simulink model "CrazyClover_Velocity_control"  (R2020b)
settings: Solver=VariableStepAuto  StartTime=0.0  StopTime=10.0  RelTol=1e-3
values from neighbouring files (symbols this model uses):
  controller_matrix = [mass/(4*gravity)*1000 mass/(4*gravity)*1000 mass/(4*gravity)*1000 mass/(4*gravity)*1000 ... (first row only)    [sim_param.m]
  kM1 = Armlength /sqrt(2)    [sim_param.m]
  kM2 = Armlength /sqrt(2)    [sim_param.m]
  kM3 = 1    [sim_param.m]
undefined symbols (not defined in the file or in its folder): Pitch, Pitchrate, Roll, Rollrate, Vel, Yaw, Yawrate
libraries: pid_lib x17
(part 2 of 2)

== system CrazyClover_Velocity_control/Controller/Subsystem3/Attitude PID/pitch PID ==
  u : Inport
  PID Controller1 : pid_lib/PID Controller  Controller=PID  Form=Parallel  TimeDomain=Continuous-time  UseExternalTs=off  SampleTime=-1  IntegratorMethod=Forward Euler  FilterMethod=Forward Euler  ControllerParametersSource=internal  P=0  I=Pitch.ki  D=0  UseFilter=on  N=100  TunerSelectOption=Transfer Function Based (PID Tuner App)  InitialConditionSource=internal  InitialConditionForIntegrator=0  InitialConditionForFilter=0  DifferentiatorICPrevScaledInput=0  ExternalReset=none  TrackingMode=off  Kt=1  LimitOutput=off  SatLimitsSource=internal  UpperSaturationLimit=inf  LowerSaturationLimit=-inf  LinearizeAsGain=on  AntiWindupMode=none  Kb=1  POutMin=[]  POutMax=[]  IOutMin=[]  IOutMax=[]  DOutMin=[]  DOutMax=[]  NOutMin=[]  NOutMax=[]  SumOutMin=[]  SumOutMax=[]  SaturationOutMin=[]  SaturationOutMax=[]  PParamMin=[]  PParamMax=[]  IParamMin=[]  IParamMax=[]  DParamMin=[]  DParamMax=[]  NParamMin=[]  NParamMax=[]  KbParamMin=[]  KbParamMax=[]  KtParamMin=[]  KtParamMax=[]  KbOutMin=[]  KbOutMax=[]  KtOutMin=[]  KtOutMax=[]  IntegratorOutMin=[]  IntegratorOutMax=[]  FilterOutMin=[]  FilterOutMax=[]  SumI1OutMin=[]  SumI1OutMax=[]  SumI2OutMin=[]  SumI2OutMax=[]  SumI3OutMin=[]  SumI3OutMax=[]  SumI4OutMin=[]  SumI4OutMax=[]  SumDOutMin=[]  SumDOutMax=[]  DifferentiatorOutMin=[]  DifferentiatorOutMax=[]  FilterDiffOutCoefMin=[]  FilterDiffOutCoefMax=[]  ReciprocalOutMin=[]  ReciprocalOutMax=[]  SumDenOutMin=[]  SumDenOutMax=[]  SumNumOutMin=[]  SumNumOutMax=[]  DivideOutMin=[]  DivideOutMax=[]  UdiffTsProdOutMin=[]  UdiffTsProdOutMax=[]  NTsProdOutMin=[]  NTsProdOutMax=[]  UintegralTsProdOutMin=[]  UintegralTsProdOutMax=[]  UngainTsProdOutMin=[]  UngainTsProdOutMax=[]  IntegratorContinuousStateAttributes=''  IntegratorStateMustResolveToSignalObject=off  IntegratorRTWStateStorageClass=Auto  FilterContinuousStateAttributes=''  FilterStateMustResolveToSignalObject=off  FilterRTWStateStorageClass=Auto  ParallelPVariant=InternalParameters  IdealPVariant=Disabled  IVariant=InternalParameters  DVariant=InternalParameters  IntegratorVariant=Continuous  SatVariant=Disabled  AWVariant=Passthrough  PCopyVariant=Disabled  TRVariant=Disabled  FdbkBlocksVariant=Forward  IdealPFdbkVariant=Disabled  SatFdbkVariant=Disabled  DerivativeFilterVariant=ContFilter  NVariant=InternalParameters  NCopyVariant=Disabled  FilterICVariant=InternalICsFilter  IntegratorICVariant=InternalICs  ExternalResetVariant=Disabled  TRSumVariant=Passthrough  SumFdbkVariant=Disabled  SumVariant=Sum_PID  TsampFilterVariant=InternalTs  TsampNgainVariant=Passthrough  TsampIntegralVariant=Passthrough  ExternalSaturationOutDataTypeStr=Inherit: Same as second input
  PID Controller2 : pid_lib/PID Controller  Controller=PID  Form=Parallel  TimeDomain=Continuous-time  UseExternalTs=off  SampleTime=-1  IntegratorMethod=Forward Euler  FilterMethod=Forward Euler  ControllerParametersSource=internal  P=Pitch.kp  I=0  D=0  UseFilter=on  N=100  TunerSelectOption=Transfer Function Based (PID Tuner App)  InitialConditionSource=internal  InitialConditionForIntegrator=0  InitialConditionForFilter=0  DifferentiatorICPrevScaledInput=0  ExternalReset=none  TrackingMode=off  Kt=1  LimitOutput=off  SatLimitsSource=internal  UpperSaturationLimit=inf  LowerSaturationLimit=-inf  LinearizeAsGain=on  AntiWindupMode=none  Kb=1  POutMin=[]  POutMax=[]  IOutMin=[]  IOutMax=[]  DOutMin=[]  DOutMax=[]  NOutMin=[]  NOutMax=[]  SumOutMin=[]  SumOutMax=[]  SaturationOutMin=[]  SaturationOutMax=[]  PParamMin=[]  PParamMax=[]  IParamMin=[]  IParamMax=[]  DParamMin=[]  DParamMax=[]  NParamMin=[]  NParamMax=[]  KbParamMin=[]  KbParamMax=[]  KtParamMin=[]  KtParamMax=[]  KbOutMin=[]  KbOutMax=[]  KtOutMin=[]  KtOutMax=[]  IntegratorOutMin=[]  IntegratorOutMax=[]  FilterOutMin=[]  FilterOutMax=[]  SumI1OutMin=[]  SumI1OutMax=[]  SumI2OutMin=[]  SumI2OutMax=[]  SumI3OutMin=[]  SumI3OutMax=[]  SumI4OutMin=[]  SumI4OutMax=[]  SumDOutMin=[]  SumDOutMax=[]  DifferentiatorOutMin=[]  DifferentiatorOutMax=[]  FilterDiffOutCoefMin=[]  FilterDiffOutCoefMax=[]  ReciprocalOutMin=[]  ReciprocalOutMax=[]  SumDenOutMin=[]  SumDenOutMax=[]  SumNumOutMin=[]  SumNumOutMax=[]  DivideOutMin=[]  DivideOutMax=[]  UdiffTsProdOutMin=[]  UdiffTsProdOutMax=[]  NTsProdOutMin=[]  NTsProdOutMax=[]  UintegralTsProdOutMin=[]  UintegralTsProdOutMax=[]  UngainTsProdOutMin=[]  UngainTsProdOutMax=[]  IntegratorContinuousStateAttributes=''  IntegratorStateMustResolveToSignalObject=off  IntegratorRTWStateStorageClass=Auto  FilterContinuousStateAttributes=''  FilterStateMustResolveToSignalObject=off  FilterRTWStateStorageClass=Auto  ParallelPVariant=InternalParameters  IdealPVariant=Disabled  IVariant=InternalParameters  DVariant=InternalParameters  IntegratorVariant=Continuous  SatVariant=Disabled  AWVariant=Passthrough  PCopyVariant=Disabled  TRVariant=Disabled  FdbkBlocksVariant=Forward  IdealPFdbkVariant=Disabled  SatFdbkVariant=Disabled  DerivativeFilterVariant=ContFilter  NVariant=InternalParameters  NCopyVariant=Disabled  FilterICVariant=InternalICsFilter  IntegratorICVariant=InternalICs  ExternalResetVariant=Disabled  TRSumVariant=Passthrough  SumFdbkVariant=Disabled  SumVariant=Sum_PID  TsampFilterVariant=InternalTs  TsampNgainVariant=Passthrough  TsampIntegralVariant=Passthrough  ExternalSaturationOutDataTypeStr=Inherit: Same as second input
  Saturation : Saturate  UpperLimit=Pitch.intupper  LowerLimit=Pitch.intlower
  Scope : Scope  NumInputPorts=2
  Sum : Sum  Inputs=|++
  y : Outport
  wires:
  Saturation/1 -> Scope/1, Sum/2
  PID Controller1/1 -> Saturation/1, Scope/2
  Sum/1 -> y/1
  u/1 -> PID Controller2/1, PID Controller1/1
  PID Controller2/1 -> Sum/1

== system CrazyClover_Velocity_control/Controller/Subsystem3/Attitude PID/roll PID ==
  u : Inport
  PID Controller1 : pid_lib/PID Controller  Controller=PID  Form=Parallel  TimeDomain=Continuous-time  UseExternalTs=off  SampleTime=-1  IntegratorMethod=Forward Euler  FilterMethod=Forward Euler  ControllerParametersSource=internal  P=0  I=Roll.ki  D=0  UseFilter=on  N=100  TunerSelectOption=Transfer Function Based (PID Tuner App)  InitialConditionSource=internal  InitialConditionForIntegrator=0  InitialConditionForFilter=0  DifferentiatorICPrevScaledInput=0  ExternalReset=none  TrackingMode=off  Kt=1  LimitOutput=off  SatLimitsSource=internal  UpperSaturationLimit=inf  LowerSaturationLimit=-inf  LinearizeAsGain=on  AntiWindupMode=none  Kb=1  POutMin=[]  POutMax=[]  IOutMin=[]  IOutMax=[]  DOutMin=[]  DOutMax=[]  NOutMin=[]  NOutMax=[]  SumOutMin=[]  SumOutMax=[]  SaturationOutMin=[]  SaturationOutMax=[]  PParamMin=[]  PParamMax=[]  IParamMin=[]  IParamMax=[]  DParamMin=[]  DParamMax=[]  NParamMin=[]  NParamMax=[]  KbParamMin=[]  KbParamMax=[]  KtParamMin=[]  KtParamMax=[]  KbOutMin=[]  KbOutMax=[]  KtOutMin=[]  KtOutMax=[]  IntegratorOutMin=[]  IntegratorOutMax=[]  FilterOutMin=[]  FilterOutMax=[]  SumI1OutMin=[]  SumI1OutMax=[]  SumI2OutMin=[]  SumI2OutMax=[]  SumI3OutMin=[]  SumI3OutMax=[]  SumI4OutMin=[]  SumI4OutMax=[]  SumDOutMin=[]  SumDOutMax=[]  DifferentiatorOutMin=[]  DifferentiatorOutMax=[]  FilterDiffOutCoefMin=[]  FilterDiffOutCoefMax=[]  ReciprocalOutMin=[]  ReciprocalOutMax=[]  SumDenOutMin=[]  SumDenOutMax=[]  SumNumOutMin=[]  SumNumOutMax=[]  DivideOutMin=[]  DivideOutMax=[]  UdiffTsProdOutMin=[]  UdiffTsProdOutMax=[]  NTsProdOutMin=[]  NTsProdOutMax=[]  UintegralTsProdOutMin=[]  UintegralTsProdOutMax=[]  UngainTsProdOutMin=[]  UngainTsProdOutMax=[]  IntegratorContinuousStateAttributes=''  IntegratorStateMustResolveToSignalObject=off  IntegratorRTWStateStorageClass=Auto  FilterContinuousStateAttributes=''  FilterStateMustResolveToSignalObject=off  FilterRTWStateStorageClass=Auto  ParallelPVariant=InternalParameters  IdealPVariant=Disabled  IVariant=InternalParameters  DVariant=InternalParameters  IntegratorVariant=Continuous  SatVariant=Disabled  AWVariant=Passthrough  PCopyVariant=Disabled  TRVariant=Disabled  FdbkBlocksVariant=Forward  IdealPFdbkVariant=Disabled  SatFdbkVariant=Disabled  DerivativeFilterVariant=ContFilter  NVariant=InternalParameters  NCopyVariant=Disabled  FilterICVariant=InternalICsFilter  IntegratorICVariant=InternalICs  ExternalResetVariant=Disabled  TRSumVariant=Passthrough  SumFdbkVariant=Disabled  SumVariant=Sum_PID  TsampFilterVariant=InternalTs  TsampNgainVariant=Passthrough  TsampIntegralVariant=Passthrough  ExternalSaturationOutDataTypeStr=Inherit: Same as second input
  PID Controller2 : pid_lib/PID Controller  Controller=PID  Form=Parallel  TimeDomain=Continuous-time  UseExternalTs=off  SampleTime=-1  IntegratorMethod=Forward Euler  FilterMethod=Forward Euler  ControllerParametersSource=internal  P=Roll.kp  I=0  D=0  UseFilter=on  N=100  TunerSelectOption=Transfer Function Based (PID Tuner App)  InitialConditionSource=internal  InitialConditionForIntegrator=0  InitialConditionForFilter=0  DifferentiatorICPrevScaledInput=0  ExternalReset=none  TrackingMode=off  Kt=1  LimitOutput=off  SatLimitsSource=internal  UpperSaturationLimit=inf  LowerSaturationLimit=-inf  LinearizeAsGain=on  AntiWindupMode=none  Kb=1  POutMin=[]  POutMax=[]  IOutMin=[]  IOutMax=[]  DOutMin=[]  DOutMax=[]  NOutMin=[]  NOutMax=[]  SumOutMin=[]  SumOutMax=[]  SaturationOutMin=[]  SaturationOutMax=[]  PParamMin=[]  PParamMax=[]  IParamMin=[]  IParamMax=[]  DParamMin=[]  DParamMax=[]  NParamMin=[]  NParamMax=[]  KbParamMin=[]  KbParamMax=[]  KtParamMin=[]  KtParamMax=[]  KbOutMin=[]  KbOutMax=[]  KtOutMin=[]  KtOutMax=[]  IntegratorOutMin=[]  IntegratorOutMax=[]  FilterOutMin=[]  FilterOutMax=[]  SumI1OutMin=[]  SumI1OutMax=[]  SumI2OutMin=[]  SumI2OutMax=[]  SumI3OutMin=[]  SumI3OutMax=[]  SumI4OutMin=[]  SumI4OutMax=[]  SumDOutMin=[]  SumDOutMax=[]  DifferentiatorOutMin=[]  DifferentiatorOutMax=[]  FilterDiffOutCoefMin=[]  FilterDiffOutCoefMax=[]  ReciprocalOutMin=[]  ReciprocalOutMax=[]  SumDenOutMin=[]  SumDenOutMax=[]  SumNumOutMin=[]  SumNumOutMax=[]  DivideOutMin=[]  DivideOutMax=[]  UdiffTsProdOutMin=[]  UdiffTsProdOutMax=[]  NTsProdOutMin=[]  NTsProdOutMax=[]  UintegralTsProdOutMin=[]  UintegralTsProdOutMax=[]  UngainTsProdOutMin=[]  UngainTsProdOutMax=[]  IntegratorContinuousStateAttributes=''  IntegratorStateMustResolveToSignalObject=off  IntegratorRTWStateStorageClass=Auto  FilterContinuousStateAttributes=''  FilterStateMustResolveToSignalObject=off  FilterRTWStateStorageClass=Auto  ParallelPVariant=InternalParameters  IdealPVariant=Disabled  IVariant=InternalParameters  DVariant=InternalParameters  IntegratorVariant=Continuous  SatVariant=Disabled  AWVariant=Passthrough  PCopyVariant=Disabled  TRVariant=Disabled  FdbkBlocksVariant=Forward  IdealPFdbkVariant=Disabled  SatFdbkVariant=Disabled  DerivativeFilterVariant=ContFilter  NVariant=InternalParameters  NCopyVariant=Disabled  FilterICVariant=InternalICsFilter  IntegratorICVariant=InternalICs  ExternalResetVariant=Disabled  TRSumVariant=Passthrough  SumFdbkVariant=Disabled  SumVariant=Sum_PID  TsampFilterVariant=InternalTs  TsampNgainVariant=Passthrough  TsampIntegralVariant=Passthrough  ExternalSaturationOutDataTypeStr=Inherit: Same as second input
  Saturation : Saturate  UpperLimit=Roll.intupper  LowerLimit=Roll.intlower
  Scope : Scope  NumInputPorts=2
  Sum : Sum  Inputs=|++
  y : Outport
  wires:
  PID Controller2/1 -> Sum/1
  u/1 -> PID Controller1/1, PID Controller2/1
  Sum/1 -> y/1
  PID Controller1/1 -> Scope/2, Saturation/1
  Saturation/1 -> Sum/2, Scope/1

== matlab function CrazyClover_Velocity_control/Controller/Subsystem3/velocity to attitude1 ==
  data: Vx input; Roll output; Pitch output; Vy input
function [Roll, Pitch]= fcn(Vx, Vy)

Roll = -Vy;
Pitch = +Vx;

== matlab function CrazyClover_Velocity_control/Plant/Subsystem/MATLAB Function ==
  data: R input; Rd output; Wb input
function Rd = fcn(R, Wb)
wx = Wb(1);
wy = Wb(2);
wz = Wb(3);
Wb = [ 0    -wz   wy;
       wz    0   -wx;
      -wy    wx   0];
Rd = R * Wb;

== matlab function CrazyClover_Velocity_control/Plant/actuator/pwm -> gram ==
  data: m1_pwm input; m1 output; m2_pwm input; m3_pwm input; m4_pwm input; m2 output; m3 output; m4 output
function [m1, m2,m3, m4]= func(m1_pwm, m2_pwm, m3_pwm, m4_pwm)

% F [16bit] Wddb [16bit]

% m1_pwm = moter_in(1);
% m2_pwm = moter_in(2);
% m3_pwm = moter_in(3);
% m4_pwm = moter_in(4);
m1_map = [2.1910e-07 0.0022 0];
m2_map = [2.1910e-07 0.0022 0];
m3_map = [2.1161e-07 0.0024 0];
m4_map = [2.0210e-07 0.0024 0];
% m_avs = (m1_pwm + m2_pwm + m3_pwm + m4_pwm)/4;
% m1_pwm = m_avs;
% m2_pwm = m_avs;
% m3_pwm = m_avs;
% m4_pwm = m_avs;
if m1_pwm > 0
    m1 = m1_map * [m1_pwm^2;m1_pwm;1];
else
    m1 = -m1_map * [m1_pwm^2;-m1_pwm;1];
end
if m2_pwm > 0
    m2 = m2_map * [m2_pwm^2;m2_pwm;1];
else
    m2 = -m2_map * [m2_pwm^2;-m2_pwm;1];
end
if m3_pwm > 0
    m3 = m3_map * [m3_pwm^2;m3_pwm;1];
else
    m3 = -m3_map * [m3_pwm^2;-m3_pwm;1];
end
if m1_pwm > 0
    m4 = m4_map * [m4_pwm^2;m4_pwm;1];
else
    m4 = -m4_map * [m4_pwm^2;-m4_pwm;1];
end

== matlab function CrazyClover_Velocity_control/Plant/Subsystem/MATLAB Function2 ==
  data: W input; Euler_angle_rate output; RPY input
function Euler_angle_rate = fcn(W, RPY)
roll = RPY(1);
pitch = RPY(2);
yaw = RPY(3);
rollS = sin(roll); rollC = cos(roll);           
pitchS = sin(pitch); pitchC = cos(pitch);       


Euler_angle_rate = pinv([1 0 -pitchS;
     0 rollC  pitchC * rollS;
     0 -rollS pitchC * rollC]) * W;

== matlab function CrazyClover_Velocity_control/Plant/moter map/gram->pwm1 2 ==
  data: x input; y1_invf output
function y1_invf = m1_map(x)
%#codegen

%    This function was generated by the Symbolic Math Toolbox version 8.6.
%    24-Aug-2022 00:51:31
if x > 0
    y1_invf = sqrt(x.*8.309953163553529e-7+8.77420076969215e-6).*2.406752433662037e+6-4.951128620134714e+3;
else
    x = abs(x);
    y1_invf = -(sqrt(x.*8.309953163553529e-7+8.77420076969215e-6).*2.406752433662037e+6-4.951128620134714e+3);
end

== matlab function CrazyClover_Velocity_control/Plant/Subsystem/Dynamics1 ==
  data: F input; Pdd output; M input; Wb input; R input; Wdd output
function [Pdd, Wdd]  = fcn(F, M, Wb, R)
m = 500;
e3 = [0 0 1]';
g = 9.8;

% 各加速度計算（ボディー座標系）
Pdd = 9.8 * F*R*e3/m - g*e3;
I = [1 0 0;
     0 1 0;
     0 0 1]*10^(-2);
% 各加速度計算（ボディー座標系）
Wdd = pinv(I)*(M - cross(Wb, I * Wb));

== matlab function CrazyClover_Velocity_control/Plant/moter map/gram->pwm2 ==
  data: x input; y2_invf output
function y2_invf = m2_map(x)
%#codegen

%    This function was generated by the Symbolic Math Toolbox version 8.6.
%    24-Aug-2022 00:51:31
if x > 0
    y2_invf = sqrt(x.*8.763965396891775e-7+1.033956593757182e-5).*2.282071995297151e+6-5.020028004430765e+3;
else
    x = abs(x);
    y2_invf = -(sqrt(x.*8.763965396891775e-7+1.033956593757182e-5).*2.282071995297151e+6-5.020028004430765e+3);
end

== matlab function CrazyClover_Velocity_control/Plant/moter map/gram->pwm3 ==
  data: x input; y3_invf output
function y3_invf = m3_map(x)
%#codegen

%    This function was generated by the Symbolic Math Toolbox version 8.6.
%    24-Aug-2022 00:51:31

if x > 0
    y3_invf = sqrt(x.*8.464410710967024e-7+1.206468234853723e-5).*2.362834305061159e+6-5.75446231128539e+3;
else
    x = abs(x);
    y3_invf = -(sqrt(x.*8.464410710967024e-7+1.206468234853723e-5).*2.362834305061159e+6-5.75446231128539e+3);
end

== matlab function CrazyClover_Velocity_control/Plant/moter map/gram->pwm4 ==
  data: x input; y4_invf output
function y4_invf = m4_map(x)
%#codegen

%    This function was generated by the Symbolic Math Toolbox version 8.6.
%    24-Aug-2022 00:51:31
if x > 0
    y4_invf = sqrt(x.*8.083914057959226e-7+1.102319411174238e-5).*2.474049062942287e+6-5.961111523577613e+3;
else
    x = abs(x);
    y4_invf = -(sqrt(x.*8.083914057959226e-7+1.102319411174238e-5).*2.474049062942287e+6-5.961111523577613e+3);
end

== matlab function CrazyClover_Velocity_control/Controller/Subsystem3/MATLAB Function ==
  data: RPY_ref_world input; RPY_ref_body output; yaw input
function RPY_ref_body = fcn(RPY_ref_world, yaw)

Ryaw = [cos(yaw) -sin(yaw) 0;
        sin(yaw)  cos(yaw) 0;
        0         0        1];
tmp = Ryaw * RPY_ref_world';
RPY_ref_body = [tmp(1) tmp(2) tmp(3)];
